simulink model "doc_receiverimpairments_dqpsk"  (R2014a)
settings: Solver=VariableStepDiscrete  StartTime=0.0  StopTime=inf  RelTol=1e-3
undefined symbols (not defined in the file or in its folder): commblksprivate, Info, magnitude, Newton, Raphson
libraries: dspstat3 x8, commrflib2 x6, commsink2 x4, commdigbbndpm3 x3, dspobslib x2, dspmathops x1, commrandsrc2 x1
settings Model: ExtModeAutoUpdateStatusClock=off  Creator=The MathWorks Inc.
settings DataIOCC: SignalLoggingSaveFormat=ModelDataLogs  SaveOutput=off  SaveTime=off  SignalLoggingName=sigsOut
settings OptimizationCC: BooleanDataType=off  ExpressionDepthLimit=2147483647  InitFltsAndDblsToZero=on  EfficientMapNaN2IntZero=off
settings DebuggingCC: SaveWithParameterizedLinksMsg=none  UnderspecifiedInitializationDetection=Classic  SignalResolutionControl=TryResolveAllWithWarning  SolverPrmCheckMsg=none  MultiTaskDSMMsg=warning  MultiTaskCondExecSysMsg=none  SigSpecEnsureSampleTimeMsg=none  FcnCallInpInsideContextMsg=UseLocalSettings  StateNameClashWarn=warning  StrictBusMsg=None
settings HardwareCC: TargetUnknown=on
settings RTWCC: IncludeERTFirstTime=on
settings GRTTargetCC: TargetFcnLib=ansi_tfl_tmw.mat  CombineOutputUpdateFcns=off  GRTInterface=on

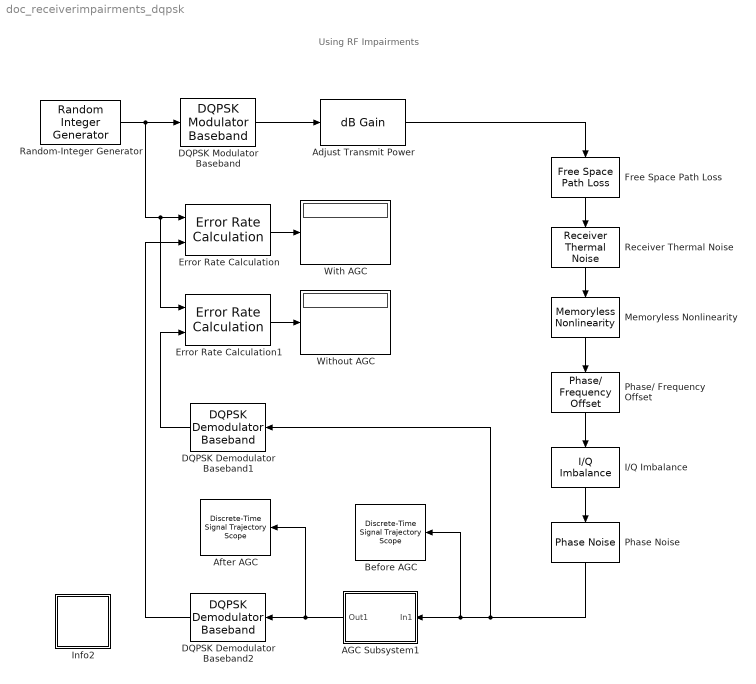
== system doc_receiverimpairments_dqpsk ==
  note: Using RF Impairments
  AGC Subsystem1 : Subsystem  mask{Pavg=1}
      mask prompts: Pavg "Average output power:"
      mask Display: disp('AGC');
  Adjust Transmit Power : dspmathops/dB Gain  dB=-73  intype=Amplitude
  After AGC : commsink2/Discrete-Time Signal Trajectory Scope  Tag=SignalTrajectory  sampPerSymb=8  offsetEye=0  numTraces=40  numNewFrames=10  LineStyles=-  LineColors=b  fading=on  render=on  AxisGrid=on  xMin=-1.14147836535369  xMax=1.13865133953243  yMin=-1.11566714554676  yMax=1.16446255933936  inphaseLabel=In-phase Amplitude  quadratureLabel=Quadrature Amplitude  openScopeAtSimStart=on  FrameNumber=off  FigPos=[65 82 367 291]  figTitle=Signal Trajectory  numLinesMax=8  block_type_=xy
  Before AGC : commsink2/Discrete-Time Signal Trajectory Scope  Tag=SignalTrajectory  sampPerSymb=8  offsetEye=0  numTraces=40  numNewFrames=10  LineStyles=-  LineColors=b  fading=on  render=on  AxisGrid=on  xMin=-1e-006  xMax=1e-006  yMin=-1e-006  yMax=1e-006  inphaseLabel=In-phase Amplitude  quadratureLabel=Quadrature Amplitude  openScopeAtSimStart=on  FrameNumber=off  FigPos=[514 89 348 283]  figTitle=Signal Trajectory  numLinesMax=8  block_type_=xy
  DQPSK Demodulator Baseband1 : commdigbbndpm3/DQPSK Demodulator Baseband  OutType=Integer  Dec=Binary  Ph=pi/4  outDtype1=double  outDtype2=double
  DQPSK Demodulator Baseband2 : commdigbbndpm3/DQPSK Demodulator Baseband  OutType=Integer  Dec=Binary  Ph=pi/4  outDtype1=double  outDtype2=double
  DQPSK Modulator Baseband : commdigbbndpm3/DQPSK Modulator Baseband  InType=Integer  Enc=Binary  Ph=pi/4  outDtype=double
  Error Rate Calculation : commsink2/Error Rate Calculation  N=0  st_delay=1000  cp_mode=Entire frame  subframe=[]  PMode=Port  WsName=ErrorVec  RsMode2=off  stop=off  numErr=100  maxBits=1e6
  Error Rate Calculation1 : commsink2/Error Rate Calculation  N=0  st_delay=1000  cp_mode=Entire frame  subframe=[]  PMode=Port  WsName=ErrorVec  RsMode2=off  stop=off  numErr=100  maxBits=1e6
  Free Space Path Loss : commrflib2/Free Space Path Loss  mode=Distance and Frequency  dB=10  d=.2  fc=900
  I/Q Imbalance : commrflib2/I//Q Imbalance  ampImbal=12  phsImbal=0  Idc=0  Qdc=0
  Info2 : Subsystem  AncestorBlock=commblksprivate/Info  mask(Info){}
      settings: OpenFcn=helpview([docroot '/toolbox/comm/comm.map'], 'doc_receiverimpairments_dqpsk')
      mask Display: disp('Info')
  Memoryless Nonlinearity : commrflib2/Memoryless Nonlinearity  model_select=Cubic polynomial  linGaindB=10  GindB=0  iip3=13  am2pm=0  LPwrLimAMPM=10  UPwrLimAMPM=inf  amam=[2.1587 1.1517]  ampm=[4.0330 9.1040]  x=[8.1081 1.5413 6.5202 -0.0718]  y=[4.6645 2.0965 10.88 -0.003]  p=0.5  GoutdB=0  vsat=1
  Phase Noise : commrflib2/Phase Noise  PhNs=-76  Fo=40  Fs=1024  seed=2137
  Phase/ Frequency Offset : commrflib2/Phase// Frequency Offset  phaseOffset=30  freqPort=off  freqOffset=2
  Random-Integer Generator : commrandsrc2/Random Integer Generator  mul=4  seed=1233  Ts=1e-4  frameBased=on  sampPerFrame=100  orient=off  outDataType=double
  Receiver Thermal Noise : commrflib2/Receiver Thermal Noise  method=Noise temperature  ntemp=290  nfigure=20  nfactor=2  seed=67987
  With AGC : Display
  Without AGC : Display
  wires:
  Random-Integer Generator/1 -> Error Rate Calculation/1, Error Rate Calculation1/1, DQPSK Modulator Baseband/1
  DQPSK Modulator Baseband/1 -> Adjust Transmit Power/1
  Free Space Path Loss/1 -> Receiver Thermal Noise/1
  Phase/ Frequency Offset/1 -> I/Q Imbalance/1
  I/Q Imbalance/1 -> Phase Noise/1
  Adjust Transmit Power/1 -> Free Space Path Loss/1
  Receiver Thermal Noise/1 -> Memoryless Nonlinearity/1
  Memoryless Nonlinearity/1 -> Phase/ Frequency Offset/1
  DQPSK Demodulator Baseband2/1 -> Error Rate Calculation/2
  AGC Subsystem1/1(Out1) -> After AGC/1, DQPSK Demodulator Baseband2/1
  Phase Noise/1 -> AGC Subsystem1/1(In1), Before AGC/1, DQPSK Demodulator Baseband1/1
  Error Rate Calculation/1 -> With AGC/1
  Error Rate Calculation1/1 -> Without AGC/1
  DQPSK Demodulator Baseband1/1 -> Error Rate Calculation1/2

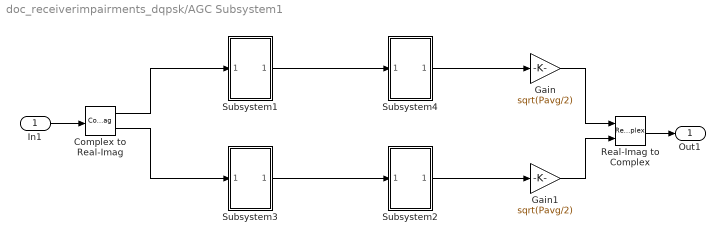
== system doc_receiverimpairments_dqpsk/AGC Subsystem1 ==
  In1 : Inport
  Complex to Real-Imag : ComplexToRealImag
  Gain : Gain  Gain=sqrt(Pavg/2)  OutDataTypeStr=Inherit: Same as input  ParamDataTypeStr=Inherit: Same as input
  Gain1 : Gain  Gain=sqrt(Pavg/2)  OutDataTypeStr=Inherit: Same as input  ParamDataTypeStr=Inherit: Same as input
  Real-Imag to Complex : RealImagToComplex
  Subsystem1 : Subsystem
  Subsystem2 : Subsystem
  Subsystem3 : Subsystem
  Subsystem4 : Subsystem
  Out1 : Outport
  wires:
  Gain/1 -> Real-Imag to Complex/1
  Subsystem2/1(Out1) -> Gain1/1
  In1/1 -> Complex to Real-Imag/1
  Gain1/1 -> Real-Imag to Complex/2
  Real-Imag to Complex/1 -> Out1/1
  Complex to Real-Imag/1 -> Subsystem1/1(In1)
  Subsystem1/1(Out1) -> Subsystem4/1(In1)
  Complex to Real-Imag/2 -> Subsystem3/1(In1)
  Subsystem3/1(Out1) -> Subsystem2/1(In1)
  Subsystem4/1(Out1) -> Gain/1

== system doc_receiverimpairments_dqpsk/Info2 ==

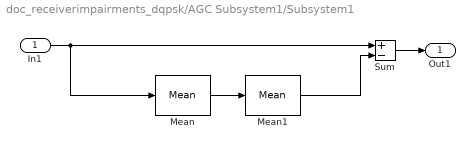
== system doc_receiverimpairments_dqpsk/AGC Subsystem1/Subsystem1 ==
  In1 : Inport
  Mean : dspstat3/Mean  run=on  reset_popup=None  InputProcessing=Columns as channels (frame based)  directionMode=Each column  dimension=1  treatSBRowAsCol=on  roiEnable=off  roiType=Rectangles  roiPortion=Entire ROI  roiOutput=Individual statistics for each ROI  roiFlag=off  outputDataTypeStr=Inherit: Same as accumulator  outputLastDataTypeStr=Inherit: Same as accumulator  outputMin=[]  outputMax=[]  roundingMode=Floor  overflowMode=off
  Mean1 : dspstat3/Mean  run=off  reset_popup=None  InputProcessing=Columns as channels (frame based)  directionMode=Each column  dimension=1  treatSBRowAsCol=on  roiEnable=off  roiType=Rectangles  roiPortion=Entire ROI  roiOutput=Individual statistics for each ROI  roiFlag=off  outputDataTypeStr=Inherit: Same as accumulator  outputLastDataTypeStr=Inherit: Same as accumulator  outputMin=[]  outputMax=[]  roundingMode=Floor  overflowMode=off
  Sum : Sum  Inputs=+-  SaturateOnIntegerOverflow=on  InputSameDT=on  OutDataTypeStr=Inherit: Same as first input
  Out1 : Outport
  wires:
  Sum/1 -> Out1/1
  In1/1 -> Sum/1, Mean/1
  Mean/1 -> Mean1/1
  Mean1/1 -> Sum/2

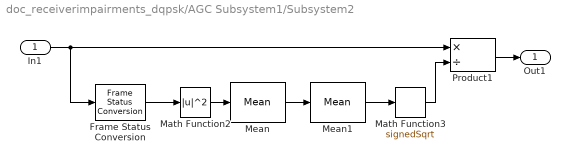
== system doc_receiverimpairments_dqpsk/AGC Subsystem1/Subsystem2 ==
  In1 : Inport
  Frame Status Conversion : dspobslib/Frame Status Conversion  growRefPort=off  outframe=Sample-based
  Math Function2 : Math  Operator=magnitude^2  SaturateOnIntegerOverflow=on
  Math Function3 : Sqrt  Operator=signedSqrt  AlgorithmType=Newton-Raphson  SaturateOnIntegerOverflow=on
  Mean : dspstat3/Mean  run=off  reset_popup=None  InputProcessing=Columns as channels (frame based)  directionMode=Each column  dimension=1  treatSBRowAsCol=on  roiEnable=off  roiType=Rectangles  roiPortion=Entire ROI  roiOutput=Individual statistics for each ROI  roiFlag=off  outputDataTypeStr=Inherit: Same as accumulator  outputLastDataTypeStr=Inherit: Same as accumulator  outputMin=[]  outputMax=[]  roundingMode=Floor  overflowMode=off
  Mean1 : dspstat3/Mean  run=on  reset_popup=None  directionMode=Each column  dimension=1  treatSBRowAsCol=on  roiEnable=off  roiType=Rectangles  roiPortion=Entire ROI  roiOutput=Individual statistics for each ROI  roiFlag=off  outputDataTypeStr=Inherit: Same as accumulator  outputLastDataTypeStr=Inherit: Same as accumulator  outputMin=[]  outputMax=[]  roundingMode=Floor  overflowMode=off
  Product1 : Product  Inputs=*/  SaturateOnIntegerOverflow=on  InputSameDT=on  OutDataTypeStr=Inherit: Same as first input
  Out1 : Outport
  wires:
  Mean/1 -> Mean1/1
  In1/1 -> Product1/1, Frame Status Conversion/1
  Math Function3/1 -> Product1/2
  Math Function2/1 -> Mean/1
  Product1/1 -> Out1/1
  Mean1/1 -> Math Function3/1
  Frame Status Conversion/1 -> Math Function2/1

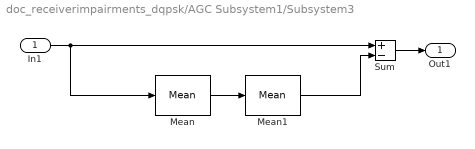
== system doc_receiverimpairments_dqpsk/AGC Subsystem1/Subsystem3 ==
  In1 : Inport
  Mean : dspstat3/Mean  run=on  reset_popup=None  InputProcessing=Columns as channels (frame based)  directionMode=Each column  dimension=1  treatSBRowAsCol=on  roiEnable=off  roiType=Rectangles  roiPortion=Entire ROI  roiOutput=Individual statistics for each ROI  roiFlag=off  outputDataTypeStr=Inherit: Same as accumulator  outputLastDataTypeStr=Inherit: Same as accumulator  outputMin=[]  outputMax=[]  roundingMode=Floor  overflowMode=off
  Mean1 : dspstat3/Mean  run=off  reset_popup=None  InputProcessing=Columns as channels (frame based)  directionMode=Each column  dimension=1  treatSBRowAsCol=on  roiEnable=off  roiType=Rectangles  roiPortion=Entire ROI  roiOutput=Individual statistics for each ROI  roiFlag=off  outputDataTypeStr=Inherit: Same as accumulator  outputLastDataTypeStr=Inherit: Same as accumulator  outputMin=[]  outputMax=[]  roundingMode=Floor  overflowMode=off
  Sum : Sum  Inputs=+-  SaturateOnIntegerOverflow=on  InputSameDT=on  OutDataTypeStr=Inherit: Same as first input
  Out1 : Outport
  wires:
  Mean1/1 -> Sum/2
  Mean/1 -> Mean1/1
  In1/1 -> Mean/1, Sum/1
  Sum/1 -> Out1/1

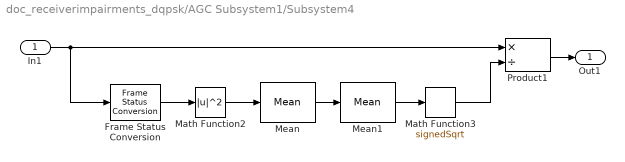
== system doc_receiverimpairments_dqpsk/AGC Subsystem1/Subsystem4 ==
  In1 : Inport
  Frame Status Conversion : dspobslib/Frame Status Conversion  growRefPort=off  outframe=Sample-based
  Math Function2 : Math  Operator=magnitude^2  SaturateOnIntegerOverflow=on
  Math Function3 : Sqrt  Operator=signedSqrt  AlgorithmType=Newton-Raphson  SaturateOnIntegerOverflow=on
  Mean : dspstat3/Mean  run=off  reset_popup=None  InputProcessing=Columns as channels (frame based)  directionMode=Each column  dimension=1  treatSBRowAsCol=on  roiEnable=off  roiType=Rectangles  roiPortion=Entire ROI  roiOutput=Individual statistics for each ROI  roiFlag=off  outputDataTypeStr=Inherit: Same as accumulator  outputLastDataTypeStr=Inherit: Same as accumulator  outputMin=[]  outputMax=[]  roundingMode=Floor  overflowMode=off
  Mean1 : dspstat3/Mean  run=on  reset_popup=None  directionMode=Each column  dimension=1  treatSBRowAsCol=on  roiEnable=off  roiType=Rectangles  roiPortion=Entire ROI  roiOutput=Individual statistics for each ROI  roiFlag=off  outputDataTypeStr=Inherit: Same as accumulator  outputLastDataTypeStr=Inherit: Same as accumulator  outputMin=[]  outputMax=[]  roundingMode=Floor  overflowMode=off
  Product1 : Product  Inputs=*/  SaturateOnIntegerOverflow=on  InputSameDT=on  OutDataTypeStr=Inherit: Same as first input
  Out1 : Outport
  wires:
  Mean1/1 -> Math Function3/1
  Product1/1 -> Out1/1
  Math Function2/1 -> Mean/1
  Math Function3/1 -> Product1/2
  In1/1 -> Product1/1, Frame Status Conversion/1
  Mean/1 -> Mean1/1
  Frame Status Conversion/1 -> Math Function2/1
